simulink model "kernal4s"  (R2015b)
settings: Solver=VariableStepAuto  StartTime=0.0  StopTime=10.0  RelTol=1e-3
values from neighbouring files (symbols this model uses):
  f51 = ([      t(0+1),t(15+1); t(16+1),t(1+1); t(2+1),t(17+1);      t(18+1),t(3+1); t(4+1),t(19+1); t(20+1),t(5+1);      t(6+1),t(21+1); t(22+1),t(7+1); t(8+1),t(23+1);      t(24+1),t(9+1); t(10+1),t(25+1); t(26+1),t(11+1);      t(12+1),t(27+1); t(28+1),t(13+1); t(14+1),t(29+1);      ])    [primefactor30.m]
settings Model: Creator=T0109428  LastModifiedBy=T0109428

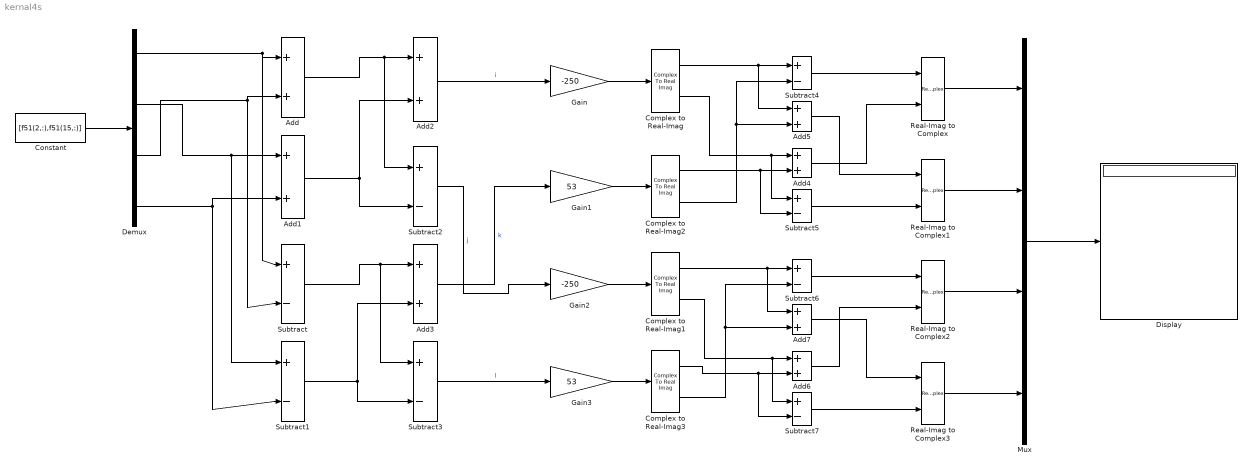
== system kernal4s ==
  Add{,1..7} (8 alike) : Sum
  Complex to Real-Imag{,1..3} (4 alike) : ComplexToRealImag
  Constant : Constant  Value=[f51(2,:),f51(15,:)]
  Demux : Demux
  Display : Display
  Gain : Gain  Gain=-250
  Gain1 : Gain  Gain=53
  Gain2 : Gain  Gain=-250
  Gain3 : Gain  Gain=53
  Mux : Mux
  Real-Imag to Complex{,1..3} (4 alike) : RealImagToComplex
  Subtract{,1..7} (8 alike) : Sum  Inputs=+-
  wires:
  Constant/1 -> Demux/1
  Demux/1 -> Subtract/1, Add/1
  Demux/3 -> Subtract/2, Add/2
  Demux/2 -> Subtract1/1, Add1/1
  Demux/4 -> Subtract1/2, Add1/2
  Add/1 -> Subtract2/1, Add2/1
  Add1/1 -> Subtract2/2, Add2/2
  Subtract/1 -> Subtract3/1, Add3/1
  Subtract1/1 -> Subtract3/2, Add3/2
  Add2/1 -> Gain/1  "i"
  Subtract2/1 -> Gain2/1  "j"
  Add3/1 -> Gain1/1  "k"
  Subtract3/1 -> Gain3/1  "l"
  Gain/1 -> Complex to Real-Imag/1
  Gain3/1 -> Complex to Real-Imag3/1
  Gain1/1 -> Complex to Real-Imag2/1
  Gain2/1 -> Complex to Real-Imag1/1
  Complex to Real-Imag/1 -> Add5/1, Subtract4/1
  Complex to Real-Imag2/2 -> Add5/2, Subtract4/2
  Subtract4/1 -> Real-Imag to Complex/1
  Complex to Real-Imag/2 -> Subtract5/1, Add4/1
  Complex to Real-Imag2/1 -> Subtract5/2, Add4/2
  Add4/1 -> Real-Imag to Complex/2
  Add5/1 -> Real-Imag to Complex1/1
  Subtract5/1 -> Real-Imag to Complex1/2
  Complex to Real-Imag1/1 -> Add7/1, Subtract6/1
  Complex to Real-Imag3/2 -> Add7/2, Subtract6/2
  Complex to Real-Imag1/2 -> Subtract7/1, Add6/1
  Complex to Real-Imag3/1 -> Subtract7/2, Add6/2
  Subtract6/1 -> Real-Imag to Complex2/1
  Add7/1 -> Real-Imag to Complex3/1
  Subtract7/1 -> Real-Imag to Complex3/2
  Add6/1 -> Real-Imag to Complex2/2
  Real-Imag to Complex3/1 -> Mux/4
  Real-Imag to Complex2/1 -> Mux/3
  Real-Imag to Complex1/1 -> Mux/2
  Real-Imag to Complex/1 -> Mux/1
  Mux/1 -> Display/1
